simulink model "Utkarsh_2005574_W3_P2"  (R2020b)
settings: Solver=FixedStepDiscrete  StartTime=0.0  StopTime=150  FixedStep=0.1  RelTol=1e-3
undefined symbols (not defined in the file): DiscIntNeverNeededParam
libraries: simulink x1
settings Model: Creator=home  LastModifiedBy=home

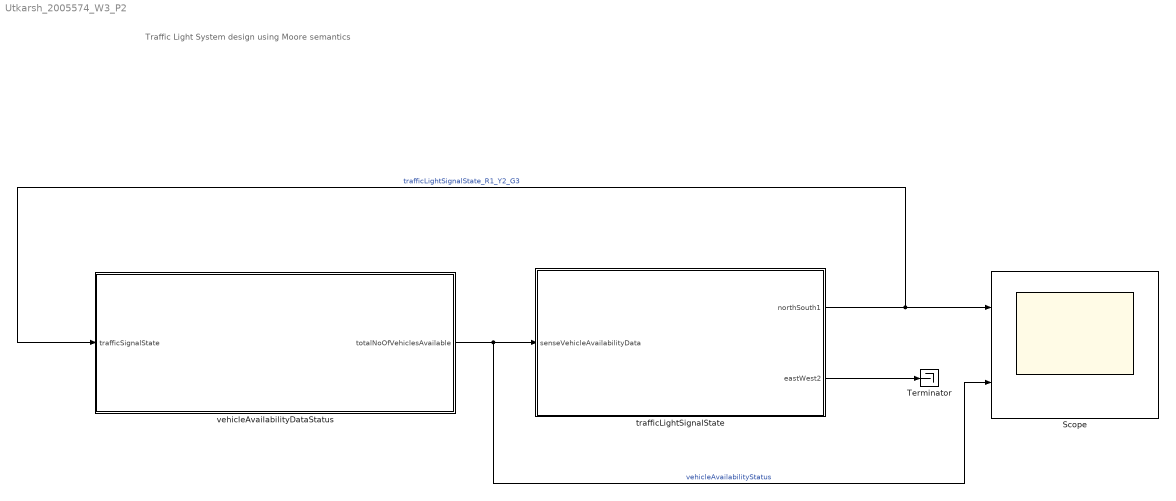
== system Utkarsh_2005574_W3_P2 ==
  note: Traffic Light System design using Moore semantics
  Scope : Scope  NumInputPorts=2
  Terminator : Terminator
  trafficLightSignalState : Stateflow chart  TreatAsAtomicUnit=on
  vehicleAvailabilityDataStatus : Subsystem
  wires:
  vehicleAvailabilityDataStatus/1(totalNoOfVehiclesAvailable) -> trafficLightSignalState/1(senseVehicleAvailabilityData), Scope/2  "vehicleAvailabilityStatus"
  trafficLightSignalState/2(eastWest2) -> Terminator/1
  trafficLightSignalState/1(northSouth1) -> vehicleAvailabilityDataStatus/1(trafficSignalState), Scope/1  "trafficLightSignalState_R1_Y2_G3"

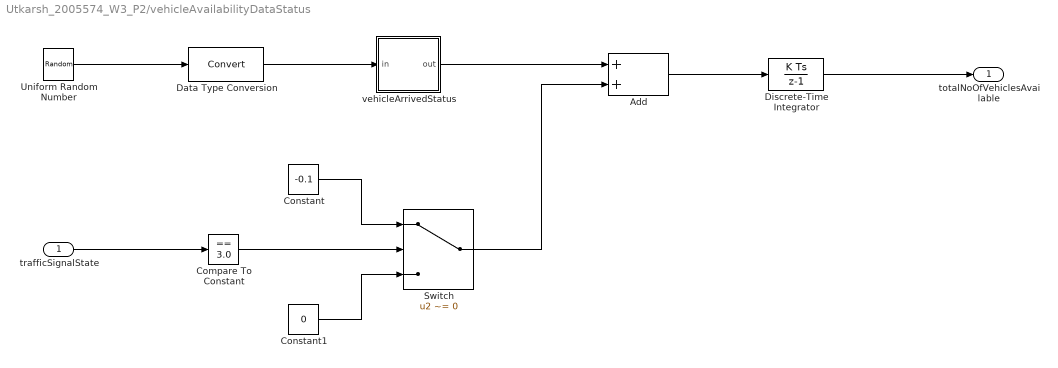
== system Utkarsh_2005574_W3_P2/vehicleAvailabilityDataStatus ==
  trafficSignalState : Inport
  Add : Sum
  Compare To Constant : simulink/Logic and Bit Operations/Compare To Constant  relop===  const=3.0  OutDataTypeStr=boolean
  Constant : Constant  Value=-0.1
  Constant1 : Constant  Value=0
  Data Type Conversion : DataTypeConversion
  Discrete-Time Integrator : DiscreteIntegrator  SampleTime=-1  LimitOutput=on  LowerSaturationLimit=0  ICPrevOutput=DiscIntNeverNeededParam  ICPrevScaledInput=DiscIntNeverNeededParam
  Switch : Switch  Criteria=u2 ~= 0
  Uniform Random Number : UniformRandomNumber  Minimum=0  Maximum=100  Seed=177836  SampleTime=0
  vehicleArrivedStatus : Stateflow chart  TreatAsAtomicUnit=on
  totalNoOfVehiclesAvailable : Outport
  wires:
  Add/1 -> Discrete-Time Integrator/1
  vehicleArrivedStatus/1(out) -> Add/1
  Switch/1 -> Add/2
  Uniform Random Number/1 -> Data Type Conversion/1
  Discrete-Time Integrator/1 -> totalNoOfVehiclesAvailable/1
  Data Type Conversion/1 -> vehicleArrivedStatus/1(in)
  Compare To Constant/1 -> Switch/2
  Constant/1 -> Switch/1
  Constant1/1 -> Switch/3
  trafficSignalState/1 -> Compare To Constant/1

== stateflow chart Utkarsh_2005574_W3_P2/vehicleAvailabilityDataStatus/vehicleArrivedStatus ==
  (default) -> (junction 7) : {out = in > 98;}
  data: in input int8; out output double

== stateflow chart Utkarsh_2005574_W3_P2/trafficLightSignalState ==
  state initialStandsill
    northSouth1=red;
    eastWest2=green;
  state haltSignalForMovingTraffic
    northSouth1=yellow;
    eastWest2=red;
  state haltForTraffic
    northSouth1=red;
    eastWest2=green;
  state moveSignalForHaltTraffic
    northSouth1=green;
    eastWest2=red
  state haltTrafficToBeReady
    northSouth1=red;
    eastWest2=yellow;
  (default) -> initialStandsill
  initialStandsill -> haltForTraffic : after(20, tick)
  haltSignalForMovingTraffic -> initialStandsill : after(3, tick)
  moveSignalForHaltTraffic -> haltSignalForMovingTraffic : after(10, tick)
  haltForTraffic -> haltTrafficToBeReady : [senseVehicleAvailabilityData]
  haltTrafficToBeReady -> moveSignalForHaltTraffic : after(3, tick)
  data: northSouth1 output; senseVehicleAvailabilityData input; eastWest2 output; red constant double =1; yellow constant double =2; green constant double =3
